simulink model "tut03_1"  (R2022a)
settings: Solver=VariableStepAuto  StartTime=0.0  StopTime=20.0  RelTol=1e-3
settings Model: Creator=vpetrone  LastModifiedBy=vpetrone

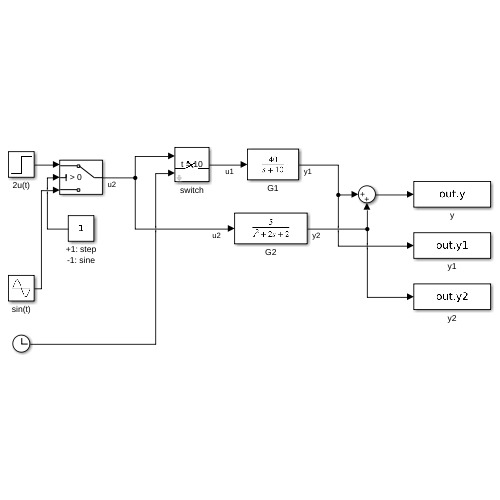
[thumbnail: Simulink's stored preview of the top-level diagram]
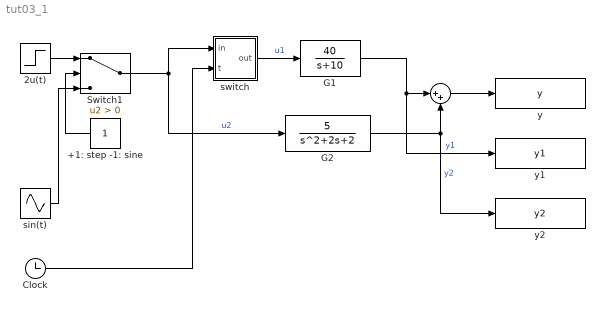
== system tut03_1 ==
  " " : Sum  Inputs=|++
  +1: step -1: sine : Constant
  2u(t) : Step  Time=0  After=2  SampleTime=0
  Clock : Clock
  G1 : TransferFcn  Numerator=[40]  Denominator=[1 10]
  G2 : TransferFcn  Numerator=[5]  Denominator=[1 2 2]
  Switch1 : Switch  Criteria=u2 > Threshold  SaturateOnIntegerOverflow=off  InputSameDT=off
  sin(t) : Sin  SampleTime=0
  switch : Subsystem  mask{T=10}
      mask prompts: T "opening_time"
      mask Display:
      | image('/home/vpetrone/Documents/MATLAB/MATLAB-Drive/FCA/simulink/assets/switch.png'); % Use "Edit Image" on toolstrip to change.
      | TT = get_param(gcb, 'opening_time');
      | disp(['t = ' TT])
  y : ToWorkspace  VariableName=y  SaveFormat=Timeseries  SampleTime=-1
  y1 : ToWorkspace  VariableName=y1  SaveFormat=Timeseries  SampleTime=-1
  y2 : ToWorkspace  VariableName=y2  SaveFormat=Timeseries  SampleTime=-1
  wires:
  G1/1 -> y1/1, " "/1  "y1"
  G2/1 -> y2/1, " "/2  "y2"
  " "/1 -> y/1
  2u(t)/1 -> Switch1/1
  sin(t)/1 -> Switch1/3
  +1: step -1: sine/1 -> Switch1/2
  Switch1/1 -> switch/1(in), G2/1  "u2"
  switch/1(out) -> G1/1  "u1"
  Clock/1 -> switch/2(t)

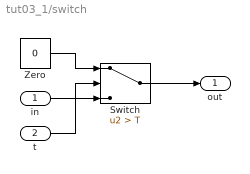
== system tut03_1/switch ==
  in : Inport
  t : Inport  Port=2
  Switch : Switch  Criteria=u2 > Threshold  Threshold=T  SaturateOnIntegerOverflow=off  InputSameDT=off
  Zero : Constant  Value=0  OutDataTypeStr=Inherit: Inherit via back propagation
  out : Outport
  wires:
  Zero/1 -> Switch/1
  Switch/1 -> out/1
  in/1 -> Switch/3
  t/1 -> Switch/2
